simulink model "Lab3"  (R2017b)
settings: Solver=VariableStepAuto  StartTime=0.0  StopTime=10  MinStep=1e-5  RelTol=1e-3  EnableMultiTasking=on
libraries: commutil2 x4, commsrccod2 x2, dspquant2 x2, dspvision x1, dspobslib x1
settings Model: Creator=pc  LastModifiedBy=Laura
settings DataIOCC: LimitDataPoints=on
settings OptimizationCC: LifeSpan=inf
settings DebuggingCC: AllowSymbolicDim=off  SFUnexpectedBacktrackingDiag=warning  SFNoUnconditionalDefaultTransitionDiag=warning  SFExecutionAtInitializationDiag=none
settings ModelReferenceCC: PropagateSignalLabelsOutOfModel=off
settings CodeAppCC: StateflowObjectComments=on
settings GRTTargetCC: TargetLangStandard=C89/C90 (ANSI)
settings ConfigComp: CovMetricSettings=dw  CovHtmlReporting=on  CovSaveCumulativeToWorkspaceVar=on  CovSaveSingleToWorkspaceVar=on  CovExternalEMLEnable=off

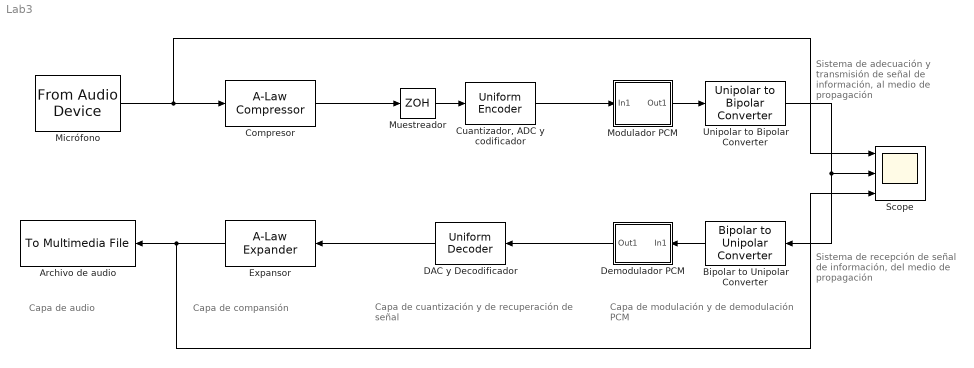
== system Lab3 ==
  note: Capa de audio
  note: Capa de compansión
  note: Capa de cuantización y
      | de recuperación de señal
  note: Sistema de adecuación y
      | transmisión de señal de
      | información, al medio de
      | propagación
  note: Capa de modulación y de
      | demodulación PCM
  note: Sistema de recepción de
      | señal de información, del
      | medio de propagación
  Archivo de audio : dspvision/To Multimedia File  outputFilename=D:\Documents\Ing. Electrónica\Comunicaciones II\Lab\Lab3\Sistema de comunicaciones\Sonido.wav  streamSelection=Audio only  videoCompressor=None (uncompressed)  audioCompressor=None (uncompressed)  imagePorts=Separate color signals  fileType=WAV  audioDatatype=32-bit integer  fourcc=RGB  videoQuality=75  mj2000CompFactor=10
      settings: SourceProductName=Computer Vision System Toolbox  SourceProductBaseCode=VP
  "Bipolar to Unipolar Converter " : commutil2/Bipolar to Unipolar Converter  M=2  polarity=Positive  dataType=Inherit via internal rule
      settings: SourceProductName=Communications System Toolbox  SourceProductBaseCode=CM
  Compresor : commsrccod2/A-Law Compressor  A=87.7  V=0.5
      settings: SourceProductName=Communications System Toolbox  SourceProductBaseCode=CM
  "Cuantizador, ADC y codificador" : dspquant2/Uniform Encoder  peak=0.5  bits=32  otype=Unsigned integer
      settings: SourceProductName=DSP System Toolbox
  DAC y Decodificador : dspquant2/Uniform Decoder  peak=0.5  bits=32  overflowMode=Saturate  otype=Double
      settings: SourceProductName=DSP System Toolbox  SourceProductBaseCode=DS
  Demodulador PCM : Subsystem
  Expansor : commsrccod2/A-Law Expander  A=87.7  V=0.5
      settings: SourceProductName=Communications System Toolbox  SourceProductBaseCode=CM
  Micrófono : dspobslib/From Audio Device  deviceName=Default  numChannels=1  sampleRate=44100  deviceDatatype=Determine from output data type  autoBufferSize=on  bufferSize=4096  queueDuration=10  frameSize=1  outputDatatype=double  defaultInputChannelMapping=on  inputChannelMapping=1:2  outputNumOverrunSamples=off  OutputFrames=off
      settings: SourceProductName=DSP System Toolbox  SourceProductBaseCode=DS
  Modulador PCM : Subsystem
  Muestreador : ZeroOrderHold  SampleTime=1/(64*4000)
  Scope : Scope  NumInputPorts=3
  "Unipolar to Bipolar Converter " : commutil2/Unipolar to Bipolar Converter  M=2  polarity=Positive  dataType=Inherit via internal rule
      settings: SourceProductName=Communications System Toolbox
  wires:
  Micrófono/1 -> Scope/1, Compresor/1
  Expansor/1 -> Scope/3, Archivo de audio/1
  Muestreador/1 -> "Cuantizador, ADC y codificador"/1
  Compresor/1 -> Muestreador/1
  DAC y Decodificador/1 -> Expansor/1
  "Bipolar to Unipolar Converter "/1 -> Demodulador PCM/1(In1)
  Modulador PCM/1(Out1) -> "Unipolar to Bipolar Converter "/1
  "Unipolar to Bipolar Converter "/1 -> Scope/2, "Bipolar to Unipolar Converter "/1
  "Cuantizador, ADC y codificador"/1 -> Modulador PCM/1(In1)
  Demodulador PCM/1(Out1) -> DAC y Decodificador/1

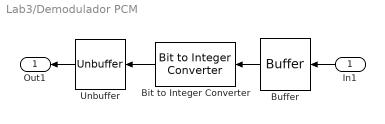
== system Lab3/Demodulador PCM ==
  In1 : Inport
  "Bit to Integer Converter " : commutil2/Bit to Integer Converter  nbits=32  bitOrder=MSB first  signedOutputValues=Unsigned  outDtype=uint32  outDtypeSigned=Inherit via internal rule
  "Buffer " : Buffer  N=32*3  OutputFrames=off
  "Unbuffer  " : Unbuffer
  Out1 : Outport
  wires:
  "Buffer "/1 -> "Bit to Integer Converter "/1
  In1/1 -> "Buffer "/1
  "Bit to Integer Converter "/1 -> "Unbuffer  "/1
  "Unbuffer  "/1 -> Out1/1

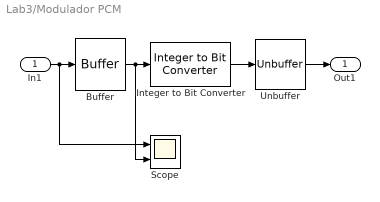
== system Lab3/Modulador PCM ==
  In1 : Inport
  "Buffer " : Buffer  N=3  OutputFrames=off
  "Integer to Bit Converter " : commutil2/Integer to Bit Converter  nbits=32  signedInputValues=Unsigned  bitOrder=MSB first  outDtype=double
  Scope : Scope  NumInputPorts=2
  "Unbuffer " : Unbuffer
  Out1 : Outport
  wires:
  "Integer to Bit Converter "/1 -> "Unbuffer "/1
  "Unbuffer "/1 -> Out1/1
  "Buffer "/1 -> Scope/2, "Integer to Bit Converter "/1
  In1/1 -> Scope/1, "Buffer "/1
